simulink model "sampleModel1524_3_sub"  (R2023a)
settings: Solver=VariableStepAuto  StartTime=0.0  StopTime=10.0  RelTol=1e-3
libraries: hdlsllib x6, simulink x2
settings Model: Creator=user1  LastModifiedBy=user1

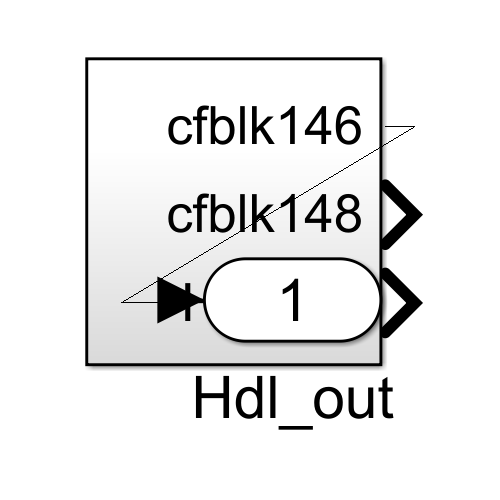
[thumbnail: Simulink's stored preview of the top-level diagram]
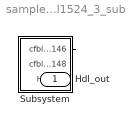
== system sampleModel1524_3_sub ==
  Subsystem : Subsystem
  Hdl_out : Outport  OutDataTypeStr=uint8
  wires:
  Subsystem/1(cfblk146) -> Hdl_out/1

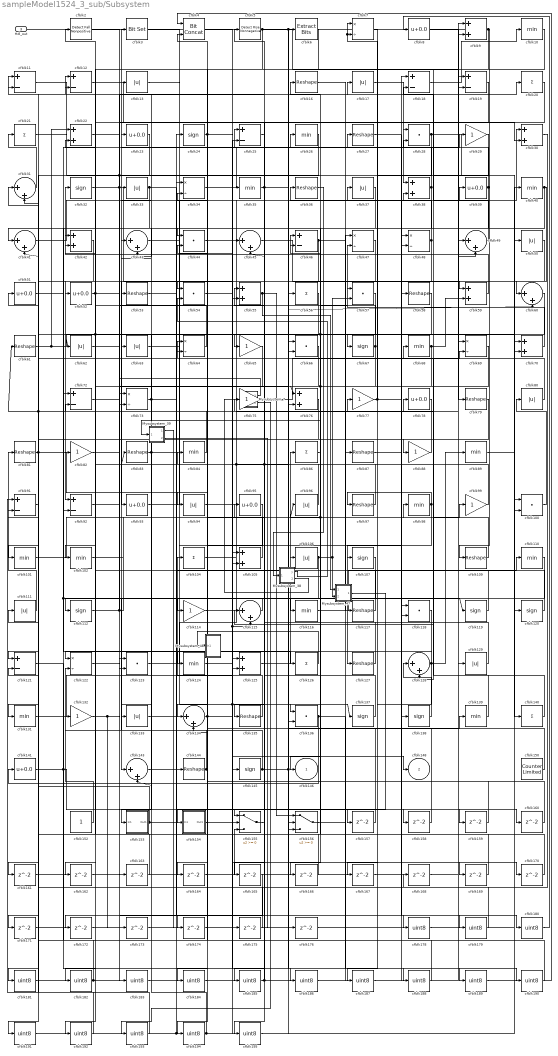
== system sampleModel1524_3_sub/Subsystem ==
  Mysubsystem_38 : Subsystem  TreatAsAtomicUnit=on  RTWFcnName=Mysubsystem_38
      settings: RTWFcnNameOpts=User specified  RTWFileNameOpts=Use function name
  Mysubsystem_39 : Subsystem  TreatAsAtomicUnit=on  RTWFcnName=Mysubsystem_39
      settings: RTWFcnNameOpts=User specified  RTWFileNameOpts=Use function name
  Mysubsystem_47 : Subsystem  TreatAsAtomicUnit=on  RTWFcnName=Mysubsystem_47
      settings: RTWFcnNameOpts=User specified  RTWFileNameOpts=Use function name
  Mysubsystem_48 : Subsystem  TreatAsAtomicUnit=on  RTWFcnName=Mysubsystem_48
      settings: RTWFcnNameOpts=User specified  RTWFileNameOpts=Use function name
  Mysubsystem_7 : Subsystem  TreatAsAtomicUnit=on  RTWFcnName=Mysubsystem_7
      settings: RTWFcnNameOpts=User specified  RTWFileNameOpts=Use function name
  cfblk{10,26,35,40,68,84,89,98,101..102,110,116,124,131,139} (15 alike) : MinMax  OutDataTypeStr=uint8
  cfblk{28,44,54,57,66,100,118,123,136} (9 alike) : DotProduct  OutDataTypeStr=uint8
  cfblk{20..21,56,86,104,126,140} (7 alike) : Sum  Inputs=+  OutDataTypeStr=uint8
  cfblk{9,22,30,38,42,55,59,70,76,105,125} (11 alike) : Sum  OutDataTypeStr=uint8
  cfblk{13,17,33,37,50,62..63,80,94,96,106,111,129,133} (14 alike) : Abs  OutDataTypeStr=uint8  SaturateOnIntegerOverflow=off
  cfblk{24,32,67,107,112,119..120,137..138,145} (10 alike) : Signum
  cfblk{16,27,36,53,58,61,79,81,83,87,97,109,117,127,135,144} (16 alike) : Reshape
  cfblk{11..12,18..19,25,46,72,91..92,121} (10 alike) : Sum  Inputs=+-  OutDataTypeStr=uint8
  cfblk{29,65,75,77,82,88,99,114,132} (9 alike) : Gain  OutDataTypeStr=uint8
  cfblk{31,41,43,45,49,60,115,128,134,143} (10 alike) : Sum  Inputs=|++  OutDataTypeStr=uint8
  cfblk{7,34,47..48,64,69,73,122} (8 alike) : Product  Inputs=*/  OutDataTypeStr=uint8  RndMeth=Zero  SaturateOnIntegerOverflow=on
  cfblk{8,23,39,51..52,78,93,95,141} (9 alike) : Bias  Bias=0.0  SaturateOnIntegerOverflow=off
  cfblk150 : hdlsllib/Sources/Counter Limited  uplimit=7  tsamp=-1
  cfblk152 : Constant  OutDataTypeStr=uint8  SampleTime=-1
  cfblk153 : Subsystem
      settings: LibrarySourceBlock=|
      | hdlsllib/Ports &
      | Subsystems/Subsystem
  cfblk154 : Subsystem
      settings: LibrarySourceBlock=|
      | hdlsllib/Ports &
      | Subsystems/Subsystem
  cfblk155 : Switch  OutDataTypeStr=uint8  SaturateOnIntegerOverflow=off  InputSameDT=off
  cfblk156 : Switch  OutDataTypeStr=uint8  SaturateOnIntegerOverflow=off  InputSameDT=off
  cfblk{157..176} (20 alike) : Delay  SampleTime=1
  cfblk{178..195} (18 alike) : DataTypeConversion  OutDataTypeStr=uint8  SaturateOnIntegerOverflow=off  RndMeth=Floor
  cfblk2 : hdlsllib/Logic and Bit Operations/Detect Fall Nonpositive  vinit=0  OutDataTypeStr=uint8
  cfblk3 : simulink/Logic and Bit Operations/Bit Set  iBit=0
      settings: LibrarySourceBlock=|
      | hdlsllib/Logic and Bit
      | Operations/Bit Set
  cfblk4 : hdlsllib/Logic and Bit Operations/Bit Concat  numInputs=2
  cfblk5 : hdlsllib/Logic and Bit Operations/Detect Rise Nonnegative  vinit=0  OutDataTypeStr=uint8
  cfblk6 : simulink/Logic and Bit Operations/Extract Bits  bitsToExtract=Upper half  numBits=8  bitIdxRange=[0 7]  outScalingMode=Preserve fixed-point scaling
      settings: LibrarySourceBlock=|
      | hdlsllib/Logic and Bit
      | Operations/Extract Bits
  cfblk146 : Outport  OutDataTypeStr=uint8  VectorParamsAs1DForOutWhenUnconnected=off
  cfblk148 : Outport  Port=2  OutDataTypeStr=uint8  VectorParamsAs1DForOutWhenUnconnected=off
  Hdl_out : Outport  Port=3  OutDataTypeStr=uint8
  wires:
  cfblk38/1 -> cfblk166/1, cfblk25/1
  cfblk42/1 -> cfblk92/1
  cfblk144/1 -> cfblk64/1, cfblk3/1
  cfblk13/1 -> cfblk136/1
  cfblk59/1 -> cfblk32/1
  cfblk98/1 -> cfblk97/1, cfblk127/1
  cfblk48/1 -> cfblk36/1, cfblk93/1
  cfblk128/1 -> cfblk187/1, cfblk124/1, cfblk89/1
  cfblk136/1 -> cfblk189/1, cfblk141/1
  cfblk135/1 -> cfblk104/1
  cfblk94/1 -> cfblk66/2, cfblk37/1
  cfblk107/1 -> cfblk143/1
  cfblk61/1 -> cfblk22/1, cfblk65/1
  cfblk41/1 -> cfblk30/1
  cfblk129/1 -> cfblk23/1
  cfblk112/1 -> cfblk57/1, cfblk98/1
  cfblk139/1 -> cfblk78/1
  cfblk137/1 -> cfblk75/1
  cfblk37/1 -> cfblk92/2
  cfblk65/1 -> cfblk153/1(In1)
  cfblk106/1 -> cfblk172/1, cfblk57/2, Mysubsystem_47/2(In2)
  cfblk86/1 -> cfblk46/1
  cfblk45/1 -> cfblk59/1
  cfblk23/1 -> cfblk52/1
  cfblk68/1 -> cfblk156/2, cfblk59/2
  cfblk3/1 -> cfblk30/2
  cfblk93/1 -> cfblk39/1
  cfblk115/1 -> cfblk114/1
  cfblk6/1 -> cfblk162/1, cfblk62/1
  cfblk58/1 -> cfblk122/1
  cfblk111/1 -> cfblk81/1
  cfblk92/1 -> cfblk17/1
  cfblk88/1 -> cfblk41/2, cfblk61/1
  cfblk120/1 -> cfblk42/1
  cfblk134/1 -> cfblk64/2, cfblk137/1, cfblk25/2
  cfblk101/1 -> cfblk45/1
  cfblk17/1 -> cfblk38/1
  cfblk110/1 -> cfblk134/1
  cfblk109/1 -> cfblk68/1
  cfblk67/1 -> cfblk184/1, cfblk16/1
  cfblk116/1 -> cfblk110/1
  cfblk33/1 -> cfblk67/1, cfblk41/1
  cfblk99/1 -> cfblk63/1
  cfblk47/1 -> cfblk131/1
  cfblk141/1 -> cfblk29/1, cfblk155/1
  cfblk9/1 -> Hdl_out/1, cfblk109/1, cfblk88/1
  cfblk150/1 -> cfblk55/1
  cfblk155/1 -> cfblk5/1
  cfblk83/1 -> cfblk143/2, cfblk138/1
  cfblk57/1 -> cfblk121/1, cfblk76/1, cfblk146/1
  cfblk70/1 -> cfblk47/2
  cfblk152/1 -> cfblk122/2
  cfblk69/1 -> cfblk112/1
  cfblk80/1 -> cfblk31/2
  cfblk118/1 -> cfblk182/1
  cfblk77/1 -> cfblk69/2, cfblk7/2, cfblk7/1
  cfblk114/1 -> cfblk77/1
  cfblk78/1 -> cfblk72/2
  cfblk22/1 -> cfblk28/1
  cfblk5/1 -> cfblk134/2, cfblk60/2, cfblk79/1
  cfblk100/1 -> cfblk80/1
  cfblk84/1 -> cfblk12/1
  cfblk91/1 -> cfblk191/1
  cfblk46/1 -> cfblk94/1, cfblk117/1
  cfblk133/1 -> cfblk34/1
  cfblk35/1 -> cfblk158/1, cfblk135/1
  cfblk50/1 -> cfblk107/1
  cfblk123/1 -> cfblk6/1
  cfblk117/1 -> cfblk84/1
  cfblk10/1 -> cfblk44/1
  cfblk34/1 -> cfblk26/1
  cfblk131/1 -> cfblk35/1
  cfblk56/1 -> cfblk194/1
  cfblk140/1 -> cfblk115/1
  cfblk51/1 -> cfblk126/1, cfblk119/1
  cfblk138/1 -> cfblk128/1
  cfblk55/1 -> cfblk156/1, Mysubsystem_47/1(In1)
  cfblk125/1 -> cfblk86/1
  cfblk32/1 -> cfblk76/2, cfblk55/2
  cfblk102/1 -> cfblk58/1
  cfblk81/1 -> cfblk51/1, cfblk144/1
  cfblk12/1 -> cfblk66/1
  cfblk127/1 -> cfblk11/1
  cfblk124/1 -> cfblk99/1
  cfblk63/1 -> cfblk38/2
  cfblk31/1 -> cfblk21/1
  cfblk96/1 -> cfblk42/2
  cfblk89/1 -> cfblk40/1
  cfblk97/1 -> cfblk45/2, cfblk83/1
  cfblk105/1 -> cfblk34/2
  cfblk39/1 -> cfblk43/2, cfblk28/2
  cfblk11/1 -> cfblk70/1
  cfblk44/1 -> cfblk156/3, cfblk115/2
  cfblk24/1 -> cfblk54/1, cfblk125/2
  cfblk16/1 -> cfblk70/2
  cfblk40/1 -> cfblk60/1, cfblk101/1
  cfblk49/1 -> cfblk18/2
  cfblk62/1 -> cfblk20/1
  cfblk43/1 -> cfblk145/1
  cfblk145/1 -> cfblk132/1, cfblk190/1, cfblk139/1
  cfblk73/1 -> cfblk116/1, cfblk13/1
  cfblk54/1 -> cfblk148/1
  cfblk52/1 -> cfblk102/1, cfblk123/1
  cfblk153/1(Out1) -> cfblk121/2, cfblk27/1
  cfblk20/1 -> cfblk82/1
  cfblk29/1 -> cfblk128/2
  cfblk18/1 -> cfblk10/1
  cfblk60/1 -> cfblk133/1
  cfblk119/1 -> cfblk96/1, Mysubsystem_39/1(In1)
  cfblk28/1 -> cfblk167/1, cfblk120/1
  cfblk104/1 -> cfblk9/1
  cfblk143/1 -> cfblk106/1
  cfblk64/1 -> cfblk2/1
  cfblk19/1 -> cfblk185/1
  cfblk75/1 -> cfblk48/1
  cfblk21/1 -> cfblk140/1, cfblk73/2
  cfblk8/1 -> cfblk49/2
  cfblk132/1 -> cfblk174/1, cfblk173/1
  cfblk7/1 -> cfblk157/1
  cfblk157/1 -> cfblk73/1
  cfblk158/1 -> cfblk18/1
  cfblk27/1 -> cfblk159/1
  cfblk159/1 -> cfblk44/2
  cfblk72/1 -> cfblk160/1
  cfblk160/1 -> cfblk47/1
  cfblk26/1 -> cfblk161/1
  cfblk161/1 -> cfblk125/1
  cfblk162/1 -> cfblk69/1
  cfblk122/1 -> cfblk163/1
  cfblk163/1 -> cfblk11/2
  cfblk95/1 -> cfblk164/1
  cfblk164/1 -> cfblk155/3
  cfblk25/1 -> cfblk165/1
  cfblk166/1 -> cfblk22/2
  cfblk167/1 -> cfblk9/2
  cfblk30/1 -> cfblk168/1
  cfblk168/1 -> cfblk49/1
  cfblk154/1(Out1) -> cfblk169/1
  cfblk169/1 -> cfblk12/2
  cfblk156/1 -> cfblk170/1
  cfblk170/1 -> cfblk46/2
  cfblk76/1 -> cfblk171/1
  cfblk171/1 -> cfblk155/2
  cfblk172/1 -> cfblk136/2
  cfblk173/1 -> cfblk43/1
  cfblk174/1 -> cfblk48/2
  cfblk175/1 -> cfblk31/1
  cfblk176/1 -> cfblk100/2
  cfblk53/1 -> cfblk178/1
  cfblk178/1 -> cfblk50/1
  cfblk2/1 -> cfblk179/1
  cfblk179/1 -> cfblk53/1
  cfblk87/1 -> cfblk180/1
  cfblk180/1 -> cfblk8/1
  cfblk79/1 -> cfblk181/1
  cfblk181/1 -> cfblk87/1
  cfblk182/1 -> cfblk72/1, cfblk105/2
  cfblk82/1 -> cfblk183/1
  cfblk183/1 -> cfblk118/1
  cfblk184/1 -> cfblk118/2
  cfblk185/1 -> cfblk129/1, cfblk95/1
  cfblk121/1 -> cfblk186/1
  cfblk186/1 -> cfblk19/1
  cfblk187/1 -> cfblk19/2
  cfblk4/1 -> cfblk188/1
  cfblk188/1 -> cfblk111/1
  cfblk189/1 -> cfblk4/1
  cfblk190/1 -> cfblk4/2
  cfblk191/1 -> cfblk24/1, cfblk105/1
  cfblk165/1 -> cfblk192/1
  cfblk192/1 -> cfblk91/1
  cfblk193/1 -> cfblk91/2
  cfblk194/1 -> cfblk100/1, cfblk33/1
  cfblk66/1 -> cfblk195/1
  cfblk195/1 -> cfblk56/1
  Mysubsystem_7/1(Out1) -> cfblk123/2
  Mysubsystem_7/2(Out2) -> cfblk193/1
  cfblk36/1 -> Mysubsystem_38/1(In1)
  Mysubsystem_38/1(y) -> cfblk54/2
  Mysubsystem_38/2(Out2) -> Mysubsystem_7/1(In1)
  Mysubsystem_39/1(Out1) -> cfblk175/1
  Mysubsystem_39/2(Out2) -> cfblk176/1
  Mysubsystem_47/1(Out1) -> cfblk154/1(In1)
  cfblk126/1 -> Mysubsystem_48/1(In1)

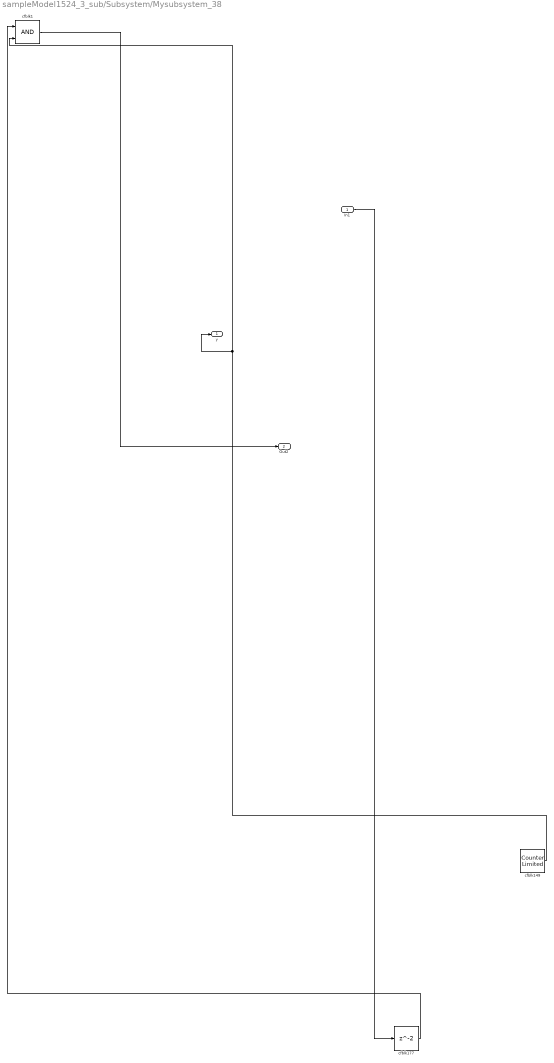
== system sampleModel1524_3_sub/Subsystem/Mysubsystem_38 ==
  In1 : Inport
  cfblk1 : Logic  AllPortsSameDT=off  OutDataTypeStr=boolean
  cfblk149 : hdlsllib/Sources/Counter Limited  uplimit=7  tsamp=-1
  cfblk177 : Delay  SampleTime=1
  y : Outport
  Out2 : Outport  Port=2
  wires:
  cfblk1/1 -> Out2/1
  In1/1 -> cfblk177/1
  cfblk177/1 -> cfblk1/1
  cfblk149/1 -> y/1, cfblk1/2

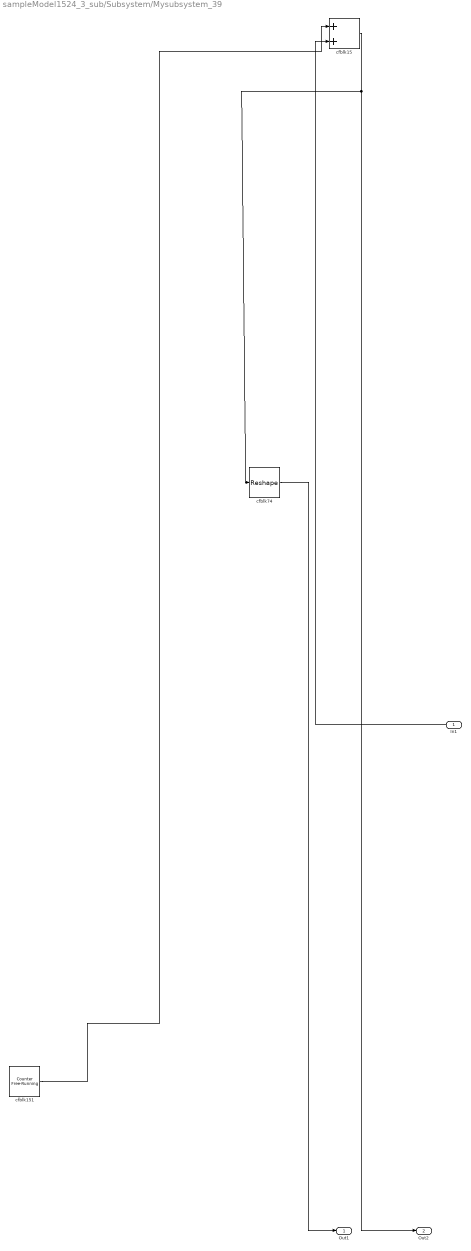
== system sampleModel1524_3_sub/Subsystem/Mysubsystem_39 ==
  In1 : Inport
  cfblk15 : Sum
  cfblk151 : hdlsllib/Sources/Counter Free-Running  NumBits=16  tsamp=-1
  cfblk74 : Reshape
  Out1 : Outport
  Out2 : Outport  Port=2
  wires:
  In1/1 -> cfblk15/2
  cfblk74/1 -> Out1/1
  cfblk151/1 -> cfblk15/1
  cfblk15/1 -> cfblk74/1, Out2/1

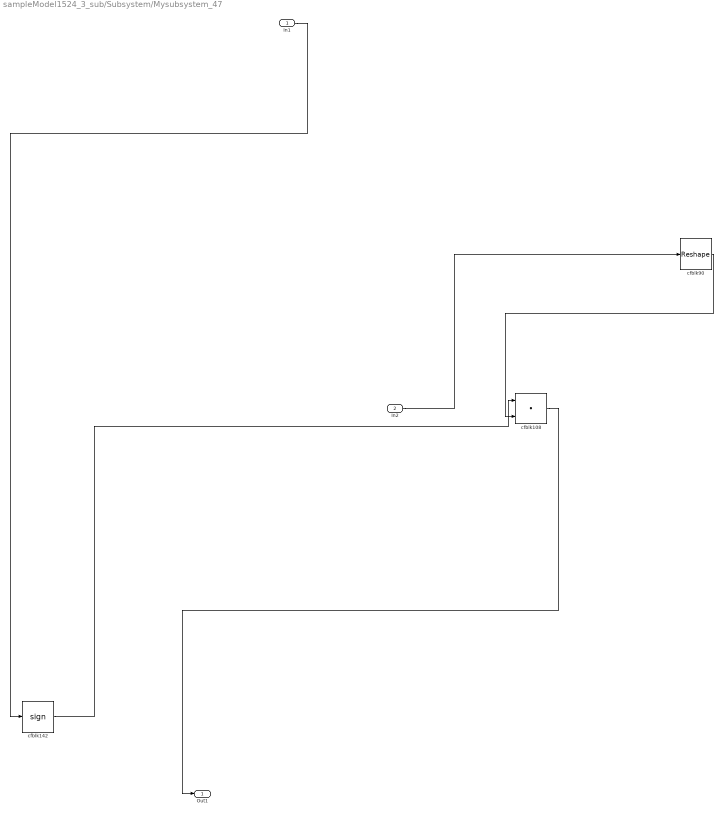
== system sampleModel1524_3_sub/Subsystem/Mysubsystem_47 ==
  In1 : Inport
  In2 : Inport  Port=2
  cfblk108 : DotProduct  OutDataTypeStr=Inherit: Inherit via internal rule
  cfblk142 : Signum
  cfblk90 : Reshape
  Out1 : Outport
  wires:
  In1/1 -> cfblk142/1
  cfblk90/1 -> cfblk108/2
  In2/1 -> cfblk90/1
  cfblk108/1 -> Out1/1
  cfblk142/1 -> cfblk108/1

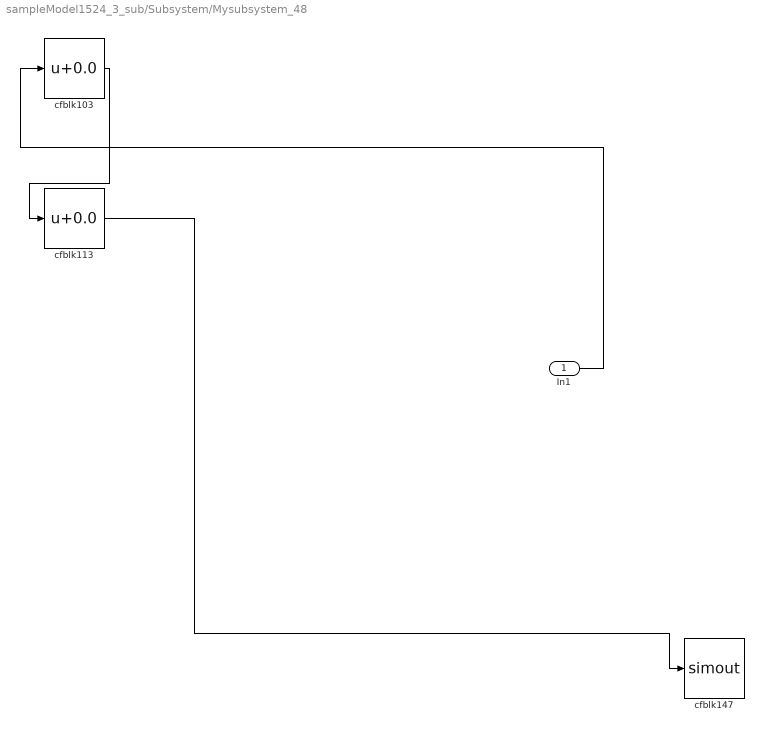
== system sampleModel1524_3_sub/Subsystem/Mysubsystem_48 ==
  In1 : Inport
  cfblk103 : Bias  Bias=0.0  SaturateOnIntegerOverflow=off
  cfblk113 : Bias  Bias=0.0  SaturateOnIntegerOverflow=off
  cfblk147 : ToWorkspace  VariableName=simout  SaveFormat=Timeseries  SampleTime=-1
  wires:
  In1/1 -> cfblk103/1
  cfblk103/1 -> cfblk113/1
  cfblk113/1 -> cfblk147/1

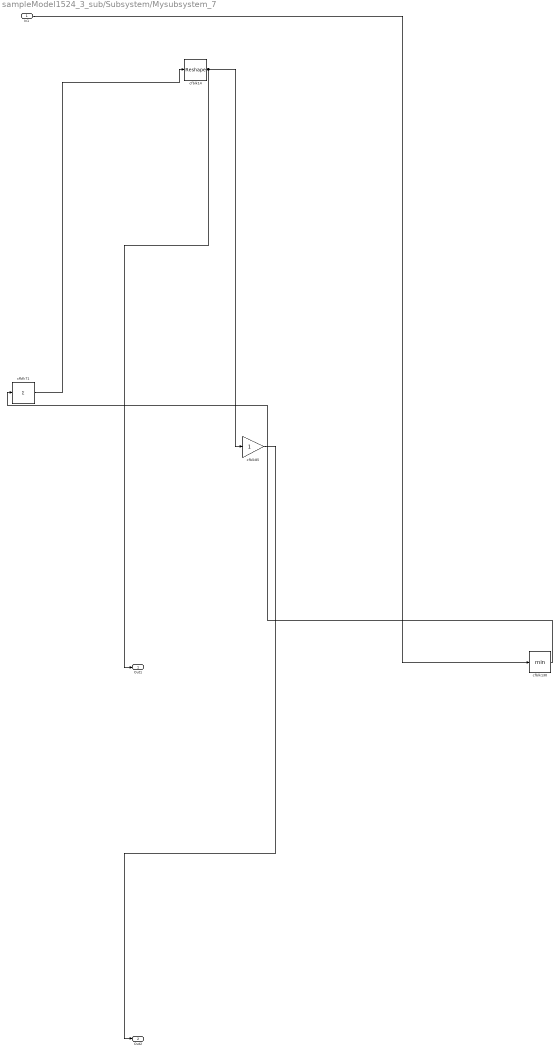
== system sampleModel1524_3_sub/Subsystem/Mysubsystem_7 ==
  In1 : Inport
  cfblk130 : MinMax
  cfblk14 : Reshape
  cfblk71 : Sum  Inputs=+
  cfblk85 : Gain
  Out1 : Outport
  Out2 : Outport  Port=2
  wires:
  cfblk14/1 -> cfblk85/1, Out1/1
  cfblk130/1 -> cfblk71/1
  In1/1 -> cfblk130/1
  cfblk71/1 -> cfblk14/1
  cfblk85/1 -> Out2/1

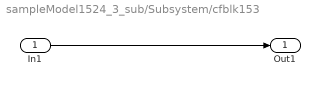
== system sampleModel1524_3_sub/Subsystem/cfblk153 ==
  In1 : Inport
  Out1 : Outport
  wires:
  In1/1 -> Out1/1

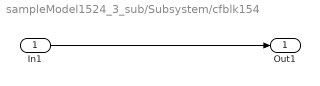
== system sampleModel1524_3_sub/Subsystem/cfblk154 ==
  In1 : Inport
  Out1 : Outport
  wires:
  In1/1 -> Out1/1
